simulink model "Control_try"  (R2021b)
settings: Solver=VariableStepAuto  StartTime=0.0  StopTime=inf  RelTol=1e-3
undefined symbols (not defined in the file or in its folder): DiscIntNeverNeededParam
libraries: mobileRoboticsLib x25, simulink_extras x1
(part 2 of 2)

== system Control_try/Team_1_behaviour/Goal_Keeper/min_Distance_Finder/Distance ==
  R_1_loc : Inport
  R_2_loc : Inport  Port=2
  Demux : Demux  Outputs=3
  Demux1 : Demux  Outputs=3
  Square : Math  Operator=square  SaturateOnIntegerOverflow=on
  Square Root : Sqrt  SaturateOnIntegerOverflow=on
  Square1 : Math  Operator=square  SaturateOnIntegerOverflow=on
  Sum : Sum  Inputs=|+-
  Sum1 : Sum  Inputs=|+-
  Sum2 : Sum  Inputs=|++
  R1_R2_dis : Outport
  wires:
  Square1/1 -> Sum2/2
  Demux/2 -> Sum1/1
  Sum2/1 -> Square Root/1
  Square/1 -> Sum2/1
  Demux/1 -> Sum/1
  Sum1/1 -> Square1/1
  Demux1/2 -> Sum1/2
  Sum/1 -> Square/1
  Demux1/1 -> Sum/2
  R_1_loc/1 -> Demux/1
  R_2_loc/1 -> Demux1/1
  Square Root/1 -> R1_R2_dis/1

== system Control_try/Team_1_behaviour/Goal_Keeper/min_Distance_Finder/Distance1 ==
  R_1_loc : Inport
  R_3_loc : Inport  Port=2
  Demux : Demux  Outputs=3
  Demux1 : Demux  Outputs=3
  Square : Math  Operator=square  SaturateOnIntegerOverflow=on
  Square Root : Sqrt  SaturateOnIntegerOverflow=on
  Square1 : Math  Operator=square  SaturateOnIntegerOverflow=on
  Sum : Sum  Inputs=|+-
  Sum1 : Sum  Inputs=|+-
  Sum2 : Sum  Inputs=|++
  R1_R3_dis : Outport
  wires:
  Square1/1 -> Sum2/2
  Demux/2 -> Sum1/1
  Sum2/1 -> Square Root/1
  Square/1 -> Sum2/1
  Demux/1 -> Sum/1
  Sum1/1 -> Square1/1
  Demux1/2 -> Sum1/2
  Sum/1 -> Square/1
  Demux1/1 -> Sum/2
  R_1_loc/1 -> Demux/1
  R_3_loc/1 -> Demux1/1
  Square Root/1 -> R1_R3_dis/1

== system Control_try/Team_1_behaviour/Goal_Keeper/min_Distance_Finder/Distance2 ==
  R_1_loc : Inport
  R_4_loc : Inport  Port=2
  Demux : Demux  Outputs=3
  Demux1 : Demux  Outputs=3
  Square : Math  Operator=square  SaturateOnIntegerOverflow=on
  Square Root : Sqrt  SaturateOnIntegerOverflow=on
  Square1 : Math  Operator=square  SaturateOnIntegerOverflow=on
  Sum : Sum  Inputs=|+-
  Sum1 : Sum  Inputs=|+-
  Sum2 : Sum  Inputs=|++
  R1_R4_dis : Outport
  wires:
  Square1/1 -> Sum2/2
  Demux/2 -> Sum1/1
  Sum2/1 -> Square Root/1
  Square/1 -> Sum2/1
  Demux/1 -> Sum/1
  Sum1/1 -> Square1/1
  Demux1/2 -> Sum1/2
  Sum/1 -> Square/1
  Demux1/1 -> Sum/2
  R_1_loc/1 -> Demux/1
  R_4_loc/1 -> Demux1/1
  Square Root/1 -> R1_R4_dis/1

== system Control_try/Team_1_behaviour/Goal_Keeper/min_Distance_Finder/R2_O_dist_val ==
  R_1_loc : Inport
  R_2_loc : Inport  Port=2
  sen_1_val : Inport  Port=3
  Chart : Stateflow chart  TreatAsAtomicUnit=on
  y : Outport
  wires:
  sen_1_val/1 -> Chart/2(sen_1_val)
  R_1_loc/1 -> Chart/1(R_1_loc)
  R_2_loc/1 -> Chart/3(R_2_loc)
  Chart/1(dist) -> y/1

== system Control_try/Team_1_behaviour/Goal_Keeper/min_Distance_Finder/R3_O_dist_val ==
  R_1_loc : Inport
  R_2_loc : Inport  Port=2
  sen_1_val : Inport  Port=3
  Chart : Stateflow chart  TreatAsAtomicUnit=on
  y : Outport
  wires:
  Chart/1(dist) -> y/1
  R_2_loc/1 -> Chart/3(R_2_loc)
  R_1_loc/1 -> Chart/1(R_1_loc)
  sen_1_val/1 -> Chart/2(sen_1_val)

== system Control_try/Team_1_behaviour/Goal_Keeper/min_Distance_Finder/R4_O_dist_val ==
  R_1_loc : Inport
  R_2_loc : Inport  Port=2
  sen_1_val : Inport  Port=3
  Chart : Stateflow chart  TreatAsAtomicUnit=on
  y : Outport
  wires:
  sen_1_val/1 -> Chart/2(sen_1_val)
  R_1_loc/1 -> Chart/1(R_1_loc)
  R_2_loc/1 -> Chart/3(R_2_loc)
  Chart/1(dist) -> y/1

== system Control_try/Team_1_behaviour/Roobot_2/min_Distance_Finder/Distance1 ==
  R_1_loc : Inport
  R_3_loc : Inport  Port=2
  Demux : Demux  Outputs=3
  Demux1 : Demux  Outputs=3
  Square : Math  Operator=square  SaturateOnIntegerOverflow=on
  Square Root : Sqrt  SaturateOnIntegerOverflow=on
  Square1 : Math  Operator=square  SaturateOnIntegerOverflow=on
  Sum : Sum  Inputs=|+-
  Sum1 : Sum  Inputs=|+-
  Sum2 : Sum  Inputs=|++
  R1_R3_dis : Outport
  wires:
  Square1/1 -> Sum2/2
  Demux/2 -> Sum1/1
  Sum2/1 -> Square Root/1
  Square/1 -> Sum2/1
  Demux/1 -> Sum/1
  Sum1/1 -> Square1/1
  Demux1/2 -> Sum1/2
  Sum/1 -> Square/1
  Demux1/1 -> Sum/2
  R_1_loc/1 -> Demux/1
  R_3_loc/1 -> Demux1/1
  Square Root/1 -> R1_R3_dis/1

== system Control_try/Team_1_behaviour/Roobot_2/min_Distance_Finder/Distance2 ==
  R_1_loc : Inport
  R_4_loc : Inport  Port=2
  Demux : Demux  Outputs=3
  Demux1 : Demux  Outputs=3
  Square : Math  Operator=square  SaturateOnIntegerOverflow=on
  Square Root : Sqrt  SaturateOnIntegerOverflow=on
  Square1 : Math  Operator=square  SaturateOnIntegerOverflow=on
  Sum : Sum  Inputs=|+-
  Sum1 : Sum  Inputs=|+-
  Sum2 : Sum  Inputs=|++
  R1_R4_dis : Outport
  wires:
  Square1/1 -> Sum2/2
  Demux/2 -> Sum1/1
  Sum2/1 -> Square Root/1
  Square/1 -> Sum2/1
  Demux/1 -> Sum/1
  Sum1/1 -> Square1/1
  Demux1/2 -> Sum1/2
  Sum/1 -> Square/1
  Demux1/1 -> Sum/2
  R_1_loc/1 -> Demux/1
  R_4_loc/1 -> Demux1/1
  Square Root/1 -> R1_R4_dis/1

== system Control_try/Team_1_behaviour/Roobot_2/min_Distance_Finder/R2_O_dist_val ==
  R_1_loc : Inport
  R_2_loc : Inport  Port=2
  sen_1_val : Inport  Port=3
  Chart : Stateflow chart  TreatAsAtomicUnit=on
  y : Outport
  wires:
  sen_1_val/1 -> Chart/2(sen_1_val)
  R_1_loc/1 -> Chart/1(R_1_loc)
  R_2_loc/1 -> Chart/3(R_2_loc)
  Chart/1(dist) -> y/1

== system Control_try/Team_1_behaviour/Roobot_2/min_Distance_Finder/R3_O_dist_val ==
  R_1_loc : Inport
  R_2_loc : Inport  Port=2
  sen_1_val : Inport  Port=3
  Chart : Stateflow chart  TreatAsAtomicUnit=on
  y : Outport
  wires:
  Chart/1(dist) -> y/1
  R_2_loc/1 -> Chart/3(R_2_loc)
  R_1_loc/1 -> Chart/1(R_1_loc)
  sen_1_val/1 -> Chart/2(sen_1_val)

== system Control_try/Team_1_behaviour/Roobot_2/min_Distance_Finder/R4_O_dist_val ==
  R_1_loc : Inport
  R_2_loc : Inport  Port=2
  sen_1_val : Inport  Port=3
  Chart : Stateflow chart  TreatAsAtomicUnit=on
  y : Outport
  wires:
  sen_1_val/1 -> Chart/2(sen_1_val)
  R_1_loc/1 -> Chart/1(R_1_loc)
  R_2_loc/1 -> Chart/3(R_2_loc)
  Chart/1(dist) -> y/1

== stateflow chart Control_try/Team 1 Behaviour/kick_direction/Chart1 ==
  state x_pos
    du:
    Vx = 1
  state x_neg
    du:
    Vx = -1
  (default) -> x_pos
  x_pos -> x_neg : [x > 0]
  x_neg -> x_pos : [x<1]
  data: Vx output; x input

== stateflow chart Control_try/Team 1 Behaviour/kick_direction/Chart2 ==
  state y_pos
    du:
    Vy = 1
  state y_neg
    du:
    Vy = -1
  (default) -> y_pos
  y_pos -> y_neg : [y > 0]
  y_neg -> y_pos : [y<1]
  data: y input; Vy output

== stateflow chart Control_try/Team 1 Behaviour/Velocity_Decider ==
  state Robot_Far
    du:
    velocity = 1;
    kick = 0;
  state Robot_Close
    du:
    velocity = 0;
    kick = 1;
  (default) -> Robot_Far
  Robot_Far -> Robot_Close : [DBR <= 0.25]
  Robot_Close -> Robot_Far : [DBR > 0.25]
  data: kick output; DBR input; velocity output

== stateflow chart Control_try/Team 1 Behaviour/Chart ==
  state second_coordinate
    du:
    actual_angle = -pi +angle + angle_bot;
  state first_coordinate
    du:
    actual_angle = angle_bot - angle;
  state ffourth_coordinate
    du:
    actual_angle = -(2*pi) + angle + angle_bot
  state Third_coordinate
    du:
    actual_angle =-(pi) - angle + angle_bot;
  (default) -> first_coordinate
  first_coordinate -> second_coordinate [order 1] : [ Rx>Bx && Ry<By ]
  second_coordinate -> first_coordinate [order 1] : [ Rx<Bx && Ry<By]
  ffourth_coordinate -> second_coordinate [order 1] : [ Rx>Bx && Ry<By ]
  first_coordinate -> Third_coordinate [order 3] : [ Rx>Bx && Ry>By]
  second_coordinate -> Third_coordinate [order 3] : [ Rx>Bx && Ry>By ]
  Third_coordinate -> second_coordinate [order 1] : [ Rx>Bx && Ry<By ]
  second_coordinate -> ffourth_coordinate [order 2] : [ Rx<Bx && Ry>By ]
  Third_coordinate -> first_coordinate [order 2] : [ Rx<Bx && Ry<By ]
  ffourth_coordinate -> first_coordinate [order 2] : [ Rx<Bx && Ry<By ]
  first_coordinate -> ffourth_coordinate [order 2] : [ Rx<Bx && Ry>By ]
  Third_coordinate -> ffourth_coordinate [order 3] : [ Rx<Bx && Ry>By ]
  ffourth_coordinate -> Third_coordinate [order 3] : [ Rx>Bx && Ry>By]
  data: Bx input; By input; Rx input; Ry input; angle input; actual_angle output; angle_bot input

== stateflow chart Control_try/Team 1 Behaviour/Chart3 ==
  state stop
    du:
    w = 0;
    v=0.25 * velocity;
  state RCW
    du:
    w = -1*1;
    v=0;
  state RCCW
    du:
    w =1*1;
    v=0;
  (default) -> stop
  stop -> RCCW [order 2] : [after(1,sec) && DT > 0]
  stop -> RCW [order 1] : [after(1,sec) && DT < 0]
  RCW -> stop [order 1] : [DT<= 0.1 && DT>= -0.1]
  RCCW -> stop [order 1] : [DT<= 0.1 && DT>= -0.1]
  RCCW -> RCW [order 2] : [DT>0]
  RCW -> RCCW [order 2] : [DT<0]
  data: velocity input; v output; DT input; w output

== stateflow chart Control_try/Referee/GOAL ==
  state Start
    en:
    right_team_goal = 0;
    left_team_goal = 0;
  state Goal_left
    en:
    right_team_goal = right_team_goal +1 ;
  state in_field
    en:
  state Goal_right
    en:
    left_team_goal = left_team_goal + 1;
  (default) -> Start
  Start -> in_field : [X > 1 && X<10 && Y > 1  && Y < 7]
  in_field -> Goal_left [order 2] : [fix(X) == 1 && Y > 2.7  && Y < 5.3 && Z < 1.2]
  Goal_right -> in_field : [X > 1 && X<10 && Y > 1  && Y < 7]
  in_field -> Goal_right [order 1] : [fix(X) == 10 && Y > 2.7  && Y < 5.3 && Z <1.2]
  Goal_left -> in_field : [X > 1 && X<10 && Y > 1  && Y < 7]
  data: X input; Y input; Z input; left_team_goal output; right_team_goal output

== stateflow chart Control_try/Referee/Throwin ==
  data: X input; Y input

== stateflow chart Control_try/Referee/Corner ==

== stateflow chart Control_try/Referee/Penelty ==

== matlab function Control_try/Enviornment/MATLAB Function ==

function plotEnvironment

coder.extrinsic('evalin');
persistent hasPlotted
if isempty(hasPlotted)
    evalin('base','environment_Plot');
    hasPlotted = true;
end

== stateflow chart Control_try/Enviornment/Ball_Dynamics/Chart ==
  state on_ground
    du:
    if(abs(F)>2.6)
    a = (abs(F)-2.6) * (F/abs(F)) / 0.43
    else
    a = 0
    end
  state off_ground
    du:
    a = F/0.43
  (default) -> on_ground
  off_ground -> on_ground : [Y ==0]
  on_ground -> off_ground : [Y > 0]
  data: Y input; F input; a output

== stateflow chart Control_try/Enviornment/Ball_Dynamics/Chart1 ==
  state calculations_neg
    du:
    vs = (abs(v))*(abs(v))*(-1)
  state calculations_pos
    du:
    vs = v*v
  (default) -> calculations_neg
  calculations_pos -> calculations_neg : [v<0]
  calculations_neg -> calculations_pos : [v>0]
  data: vs output; v input

== stateflow chart Control_try/Enviornment/Ball_Dynamics/Chart2 ==
  state on_ground
    du:
    if(abs(F)>2.6)
    a = (abs(F) - 2.6) * (F/abs(F)) / 0.43
    else
    a = 0
    end
  state off_ground
    du:
    a = F/0.43
  (default) -> on_ground
  off_ground -> on_ground : [Y ==0]
  on_ground -> off_ground : [Y > 0]
  data: Y input; F input; a output

== stateflow chart Control_try/Enviornment/Ball_Dynamics/Chart3 ==
  state calculations_neg
    du:
    vs = (abs(v))*(abs(v))*(-1)
  state calculations_pos
    du:
    vs = v*v
  (default) -> calculations_neg
  calculations_pos -> calculations_neg : [v<0]
  calculations_neg -> calculations_pos : [v>=0]
  data: vs output; v input

== stateflow chart Control_try/Enviornment/Ball_Dynamics/Chart4 ==
  state in_motion
    du:
    if (v > 0)
    a = -(0.32*0.98)
    else if(v<0)
    a = (0.32*0.98)
    end
    end
  state stationary
    du:
    a = 0;
  (default) -> in_motion
  in_motion -> stationary : [abs(v) < 0.03 | Y>0]
  stationary -> in_motion : [abs(v)>0.03]
  data: Y input; a output; v input

== stateflow chart Control_try/Team_1_behaviour/Goal_Keeper/control ==
  state Ball_Following
    du:
    kick = 0;
    if (R1_loc_Y>2.7 && R1_loc_Y<5.3)
    if(Ball_loc_Y > R1_loc_Y)
    R1_vel_Y = 0.1;
    else if (Ball_loc_Y < R1_loc_Y)
    R1_vel_Y = -0.1;
    end
    end
    else if ( R1_loc_Y > 5.3)
    R1_vel_Y = -0.1;
    else if ( R1_loc_Y < 2.7)
    R1_vel_Y = -0.1;
    end
    end
    end
  state Ball_Held
    du:
    kick = 1;
  (default) -> Ball_Following
  Ball_Following -> Ball_Held : [GB_dist < 0.25]
  Ball_Held -> Ball_Following : [GB_dist > 0.25]
  data: kick output; R1_loc_X input; Ball_loc_X input; GB_dist input; R1_loc_Y input; Ball_loc_Y input; R1_vel_Y output

== stateflow chart Control_try/Enviornment/Ball_Dynamics/Chart6 ==
  state in_motion
    du:
    if (v > 0)
    a = -(0.32*0.98)
    else if(v<0)
    a = (0.32*0.98)
    end
    end
  state stationary
    du:
    a = 0;
  (default) -> in_motion
  in_motion -> stationary : [abs(v) < 0.01 | Y>0]
  stationary -> in_motion : [abs(v)>0.02]
  data: Y input; a output; v input

== stateflow chart Control_try/Team_1_behaviour/Goal_Keeper/min_Distance_Finder/Kick_prob_calc ==
  state bot_2
    du:
    kick_direction = R_2_loc
  state bot_3
    du:
    kick_direction = R_3_loc
  state bot_4
    du:
    kick_direction = R_4_loc
  (default) -> bot_2
  bot_2 -> bot_3 [order 1] : [R1_R3_dis < R1_R2_dis && R1_R3_dis < R1_R4_dis]
  bot_3 -> bot_2 [order 1] : [R1_R2_dis < R1_R3_dis && R1_R2_dis < R1_R4_dis]
  bot_4 -> bot_2 [order 2] : [R1_R2_dis < R1_R3_dis && R1_R2_dis < R1_R4_dis]
  bot_2 -> bot_4 [order 2] : [R1_R4_dis < R1_R3_dis && R1_R4_dis < R1_R2_dis]
  bot_3 -> bot_4 [order 2] : [R1_R4_dis < R1_R3_dis && R1_R4_dis < R1_R2_dis]
  bot_4 -> bot_3 [order 1] : [R1_R3_dis < R1_R2_dis && R1_R3_dis < R1_R4_dis]
  data: R_4_loc input; R_2_loc input; R_3_loc input; R1_R2_dis input; R1_R3_dis input; R1_R4_dis input; kick_direction output

== stateflow chart Control_try/Team_1_behaviour/Goal_Keeper/min_Distance_Finder/R3_O_dist_val/Chart ==
  state calculate
    en:
    dist = 0;
    pos_x = 0;
    pos_y =0;
    dist_x =0;
    dist_y = 0;
    i=0;
    du:
    dist = 0;
    for i=1:7
    if (sen_1_val(i,3) > 4)
    pos_x = R_1_loc(1) + sen_1_val(i,1);
    pos_y = R_1_loc(2) + sen_1_val(i,2);
    dist_x = R_2_loc(1) - pos_x;
    dist_y = R_2_loc(2) - pos_y;
    dist = dist + sqrt((dist_x*dist_x) + (dist_y*dist_y));
    end
    end
  (default) -> calculate
  data: R_1_loc input; sen_1_val input; dist output; R_2_loc input; dist_y local; i local; pos_x local; pos_y local; dist_x local

== stateflow chart Control_try/Team_1_behaviour/Goal_Keeper/min_Distance_Finder/R2_O_dist_val/Chart ==
  state calculate
    en:
    dist = 0;
    pos_x = 0;
    pos_y =0;
    dist_x =0;
    dist_y = 0;
    i=0;
    du:
    dist = 0;
    for i=1:7
    if (sen_1_val(i,3) > 4)
    pos_x = R_1_loc(1) + sen_1_val(i,1);
    pos_y = R_1_loc(2) + sen_1_val(i,2);
    dist_x = R_2_loc(1) - pos_x;
    dist_y = R_2_loc(2) - pos_y;
    dist = dist + sqrt((dist_x*dist_x) + (dist_y*dist_y));
    end
    end
  (default) -> calculate
  data: R_1_loc input; sen_1_val input; dist output; R_2_loc input; dist_y local; i local; pos_x local; pos_y local; dist_x local

== stateflow chart Control_try/Team_1_behaviour/Goal_Keeper/min_Distance_Finder/R4_O_dist_val/Chart ==
  state calculate
    en:
    dist = 0;
    pos_x = 0;
    pos_y =0;
    dist_x =0;
    dist_y = 0;
    i=0;
    du:
    dist = 0;
    for i=1:7
    if (sen_1_val(i,3) > 4)
    pos_x = R_1_loc(1) + sen_1_val(i,1);
    pos_y = R_1_loc(2) + sen_1_val(i,2);
    dist_x = R_2_loc(1) - pos_x;
    dist_y = R_2_loc(2) - pos_y;
    dist = dist + sqrt((dist_x*dist_x) + (dist_y*dist_y));
    end
    end
  (default) -> calculate
  data: R_1_loc input; sen_1_val input; dist output; R_2_loc input; dist_y local; i local; pos_x local; pos_y local; dist_x local

== stateflow chart Control_try/Team_1_behaviour/Goal_Keeper/kick_direction/Chart1 ==
  state x_pos
    du:
    Vx = 1
  state x_neg
    du:
    Vx = -1
  (default) -> x_pos
  x_pos -> x_neg : [x > 0]
  x_neg -> x_pos : [x<1]
  data: Vx output; x input

== stateflow chart Control_try/Team_1_behaviour/Goal_Keeper/kick_direction/Chart2 ==
  state y_pos
    du:
    Vy = 1
  state y_neg
    du:
    Vy = -1
  (default) -> y_pos
  y_pos -> y_neg : [y > 0]
  y_neg -> y_pos : [y<1]
  data: y input; Vy output

== stateflow chart Control_try/Enviornment/kick_director/Chart ==
  state P1_kick
    du:
    KF = [p1(1);p1(2);p1(3);p1(4)]
    bot_tag = 1
  state P5_kick
    du:
    KF = p5
    bot_tag = 5
  state no_ball_kick
    du:
    KF = [0;0;0;0]
  state P2_kick
    du:
    KF = p2
    bot_tag = 2
  state P6_kick
    du:
    KF = p6
    bot_tag = 6
  state P3_kick
    du:
    KF = p3
    bot_tag = 3
  state P7_kick
    du:
    KF = p7
    bot_tag = 7
  state P4_kick
    du:
    KF = p4
    bot_tag = 4
  state P8_kick
    du:
    KF = p8
    bot_tag = 8
  (default) -> no_ball_kick
  P5_kick -> no_ball_kick : [p5(4) == 0]
  no_ball_kick -> P5_kick [order 5] : [p5(4) == 1]
  P1_kick -> no_ball_kick : [p1(4) == 0]
  no_ball_kick -> P1_kick [order 1] : [p1(4) == 1]
  no_ball_kick -> P2_kick [order 2] : [p2(4) == 1]
  no_ball_kick -> P6_kick [order 6] : [p6(4) == 1]
  P2_kick -> no_ball_kick : [p2(4) == 0]
  P6_kick -> no_ball_kick : [p6(4) == 0]
  P3_kick -> no_ball_kick : [p3(4) == 0]
  P7_kick -> no_ball_kick : [p7(4) == 0]
  no_ball_kick -> P7_kick [order 7] : [p7(4) == 1]
  no_ball_kick -> P3_kick [order 3] : [p3(4) == 1]
  no_ball_kick -> P8_kick [order 8] : [p8(4) == 1]
  no_ball_kick -> P4_kick [order 4] : [p4(4) == 1]
  P4_kick -> no_ball_kick : [p4(4) == 0]
  P8_kick -> no_ball_kick : [p8(4) == 0]
  data: bot_tag output; p1 input; p2 input; p3 input; p4 input; p5 input; p6 input; p7 input; p8 input; KF output

== matlab function Control_try/Team_1_behaviour/Goal_Keeper/min_Distance_Finder/zero_padding ==
  data: u input; y output
function y = pad(u)
% Zero-pads object detections to work with arrays of buses

y = zeros(7,3);
numElems = min(size(u,1),7);
for idx = 1:numElems
   y(idx,1:3) = u(idx,1:3); 
end
end

== matlab function Control_try/Team_1_behaviour/Goal_Keeper/MATLAB Function ==
  data: robotLoc input; newHeadingAngle output; checkpoint input
function newHeadingAngle  = ComputeHeadingAngle(robotLoc, checkpoint)

currentLocation = [robotLoc(1),robotLoc(2)];

deltaPosition = checkpoint - currentLocation;

calculatedHeadingAngle = atan2( deltaPosition(1), deltaPosition(2) );

if isnan(calculatedHeadingAngle)
    if deltaPosition(2) >= 0
        newHeadingAngle = pi/2;
    else
        newHeadingAngle = -pi/2;
    end
else
    newHeadingAngle = calculatedHeadingAngle;
end

end

== stateflow chart Control_try/Team_1_behaviour/Roobot_2/control ==
  state Ball_Following
    en,du:
    distance_to_ball = Distance(R2_loc (1), R2_loc (2), Ball_loc_X,Ball_loc_Y);
    ball_loc = [Ball_loc_X,Ball_loc_Y];
    %angle = ComputeHeadingAngle(R2_loc,ball_loc,0.05);
    [x_res, y_res] = velocityResolver(angle);
    distance_to_goal = Distance(R2_loc(1),R2_loc(2),10,4);
    if(distance_to_ball<0.15)
    pass_beh = pass_behaviour_controller(distance_to_goal,nearest_op,nearest_team);
    %kick =1;
    %else
    %move_to_ball;
    %R2_vel_X = 0.44 * x_res;
    %R2_vel_Y = 0.44 *y_res;
    %R1_vel_X = 03. * resolver(1);
    %R1_vel_Y = 0.3 * resolver(2);
    %R1_vel_X = 0.12 * resolver(1);
    %R1_vel_Y = 0.12 * resolver(2);
    end
  state Shoot
    en,du:
    distance_to_goal_1 = Distance(10,3.35,R2_loc(1),R2_loc(2));
    distance_to_goal_2 = Distance(10,4.65,R2_loc(1),R2_loc(2));
    shoot_region = shooting_spot_rev1_controller(distance_to_goal_1,GoalKeeperY,distance_to_goal_2);
    kick_angle = ComputeKickingAngle(R2_loc, [10,shoot_region]);
    kick = 1;
  state dribble
    du:
    R2_vel_X = 0;
    R2_vel_Y = 0;
  state pass
    kick_angle = ComputeKickingAngle(R2_loc, nearest_robot);
  (default) -> Ball_Following
  Shoot -> Ball_Following : [after(1,sec)]
  Ball_Following -> dribble [order 2] : [pass_beh == 2]
  dribble -> Ball_Following : [after(1,sec)]
  Ball_Following -> Shoot [order 1] : [pass_beh == 3]
  Ball_Following -> pass [order 3] : [pass_beh == 1]
  pass -> Ball_Following : [after(1,sec)]
  data: angle1 function_input; vx function_output; vy function_output; ball_distance function_input; ball_velocity function_input; movement function_output; distancetogoal function_input; nearest_oponent_distance function_input; nearest_team_player_distance function_input; pass_behaviour function_output; distance_to_goal1 function_input; goal_keeperY function_input; distance_to_goal2 function_input; centroid function_output; robotLoc function_input; checkpoint function_input; newHeadingAngle function_output; tolerance function_input; x1 function_input; y1 function_input; x2 function_input; y2 function_input; distance function_output; robotLoc function_input; checkpoint function_input; newHeadingAngle function_output; kick output; R2_loc input; Ball_loc_X input; GB_dist input; Ball_loc_Y input; R2_vel_Y output =0; ball_vel_x input; ball_vel_y input; GoalKeeperY input; distance_to_ball local; distance_to_goal_1 local; distance_to_goal_2 local; resolver local; shoot_region local; distance_to_goal local; R2_vel_X output =0; nearest_team input; nearest_team_idx input; nearest_op input; kick_angle output; pass_beh local =0; nearest_robot input; y_res local; x_res local; angle output =0; ball_loc local
  function [vx,vy] = velocityResolver(angle1):
    | function [vx,vy] = velocityResolver(angle1)
    | 
    | vx = cos(angle1);
    | vy = sin(angle1);
    | 
    | end
  function movement  = robot_moving_speed_controller(ball_distance, ball_velocity):
    | function movement  = robot_moving_speed_controller(ball_distance, ball_velocity)
    | %UNTITLED2 Summary of this function goes here
    | %   Detailed explanation goes here
    | MovingSpeedFuzzyFile= readfis('robot_moving_speed');
    | A = evalfis(MovingSpeedFuzzyFile,[ball_distance, ball_velocity]);
    | if ( A(1)<0.5 )
    | movement=1;
    | elseif ( 0.5<=A(2) && A(2)<2.5 )
    | movement=2;
    | elseif ( A(3)>2.5 )
    | movement=3;
    | end
    | 
    | end
  function pass_behaviour  = pass_behaviour_controller(distancetogoal,nearest_oponent_distance,nearest_team_player_distance):
    | function pass_behaviour  = pass_behaviour_controller(distancetogoal,nearest_oponent_distance,nearest_team_player_distance)
    | %PASS_BEHAVIOR Summary of this function goes here
    | %   Detailed explanation goes here
    | behaviourFuzzyFile= getFISCodeGenerationData('pass_behaviour.fis');
    | b = evalfis(behaviourFuzzyFile,[distancetogoal,nearest_oponent_distance,nearest_team_player_distance]);
    | 
    | if ( b<0.4 )
    | pass_behaviour=1;
    | elseif ( 0.4<=b && b<0.6 )
    | pass_behaviour=2;
    | else
    | pass_behaviour=3;
    | end
    | 
    | end
  function centroid  = shooting_spot_rev1_controller(distance_to_goal1, goal_keeperY, distance_to_goal2):
    | function centroid  = shooting_spot_rev1_controller(distance_to_goal1, goal_keeperY, distance_to_goal2)
    | %UNTITLED3 Summary of this function goes here
    | %   Detailed explanation goes here
    | ShootingSpotFuzzyFile= getFISCodeGenerationData('shooting_spot_rev1');
    | C = evalfis(ShootingSpotFuzzyFile,[distance_to_goal1, goal_keeperY, distance_to_goal2]);
    | if ( C<1 )
    | % shooting_region=1;
    | centroid = [4.65,0.3];
    | elseif ( 1<=C && C<2 )
    | % shooting_region=2;
    | centroid = [3.35,0.3];
    | elseif ( 2<=C && C<3 )
    | % shooting_region=3;
    | centroid = [4.65,0.9];
    | else
    | % shooting_region=4;
    | centroid = [3.35,0.9];
    | end
    | end
  function newHeadingAngle  = ComputeHeadingAngle(robotLoc, checkpoint,tolerance):
    | function newHeadingAngle  = ComputeHeadingAngle(robotLoc, checkpoint,tolerance)
    | 
    | currentLocation = [robotLoc(1),robotLoc(2)];
    | 
    | 
    | % Check to see if within tolerance 
    | deltaPosition = checkpoint - currentLocation;
    | distanceFromCheckpoint = norm(deltaPosition);
    | 
    | booleanAtCheckpoint = (distanceFromCheckpoint < tolerance);
    | 
    | % Calculate new heading
    | calculatedHeadingAngle = atan2( deltaPosition(2), deltaPosition(1) );
    | 
    | if isnan(calculatedHeadingAngle)
    |     if deltaPosition(2) >= 0
    |         newHeadingAngle = pi/2;
    |     else
    |         newHeadingAngle = -pi/2;
    |     end
    | else
    |     newHeadingAngle = calculatedHeadingAngle;
    | end
    | 
    | end
  function distance = Distance(x1,y1,x2,y2):
    | function distance = Distance(x1,y1,x2,y2)
    | distance = sqrt((x1-x2).^2 + (y1 +y2).^2);
    | end
  function newHeadingAngle  = ComputeKickingAngle(robotLoc, checkpoint):
    | function newHeadingAngle  = ComputeKickingAngle(robotLoc, checkpoint)
    | 
    | currentLocation = [robotLoc(1),robotLoc(2),0];
    | 
    | deltaPosition = checkpoint - currentLocation;
    | 
    | calculatedHeadingAngle = atan2( deltaPosition(2), deltaPosition(1));
    | 
    | if isnan(calculatedHeadingAngle)
    |     if deltaPosition(1) >= 0
    |         newHeadingAngle = pi/2;
    |     else
    |         newHeadingAngle = -pi/2;
    |     end
    | else
    |     newHeadingAngle = calculatedHeadingAngle;
    | end
    | 
    | end

== matlab function Control_try/Team_1_behaviour/Roobot_2/min_Distance_Finder/MATLAB Function ==
  data: min input; y output; rob3 input
function y = fcn(min, rob3)
 if min == rob3
y = 3;
 else 
     y =4;
 end
end

== stateflow chart Control_try/Team_1_behaviour/Roobot_2/min_Distance_Finder/R2_O_dist_val/Chart ==
  state calculate
    en:
    dist = 0;
    pos_x = 0;
    pos_y =0;
    dist_x =0;
    dist_y = 0;
    i=0;
    du:
    dist = 0;
    for i=1:7
    if (sen_1_val(i,3) > 4)
    pos_x = R_1_loc(1) + sen_1_val(i,1);
    pos_y = R_1_loc(2) + sen_1_val(i,2);
    dist_x = R_2_loc(1) - pos_x;
    dist_y = R_2_loc(2) - pos_y;
    dist = dist + sqrt((dist_x*dist_x) + (dist_y*dist_y));
    end
    end
  (default) -> calculate
  data: R_1_loc input; sen_1_val input; dist output; R_2_loc input; dist_y local; i local; pos_x local; pos_y local; dist_x local

== stateflow chart Control_try/Team_1_behaviour/Roobot_2/min_Distance_Finder/R3_O_dist_val/Chart ==
  state calculate
    en:
    dist = 0;
    pos_x = 0;
    pos_y =0;
    dist_x =0;
    dist_y = 0;
    i=0;
    du:
    dist = 0;
    for i=1:7
    if (sen_1_val(i,3) > 4)
    pos_x = R_1_loc(1) + sen_1_val(i,1);
    pos_y = R_1_loc(2) + sen_1_val(i,2);
    dist_x = R_2_loc(1) - pos_x;
    dist_y = R_2_loc(2) - pos_y;
    dist = dist + sqrt((dist_x*dist_x) + (dist_y*dist_y));
    end
    end
  (default) -> calculate
  data: R_1_loc input; sen_1_val input; dist output; R_2_loc input; dist_y local; i local; pos_x local; pos_y local; dist_x local

== stateflow chart Control_try/Team_1_behaviour/Roobot_2/min_Distance_Finder/R4_O_dist_val/Chart ==
  state calculate
    en:
    dist = 0;
    pos_x = 0;
    pos_y =0;
    dist_x =0;
    dist_y = 0;
    i=0;
    du:
    dist = 0;
    for i=1:7
    if (sen_1_val(i,3) > 4)
    pos_x = R_1_loc(1) + sen_1_val(i,1);
    pos_y = R_1_loc(2) + sen_1_val(i,2);
    dist_x = R_2_loc(1) - pos_x;
    dist_y = R_2_loc(2) - pos_y;
    dist = dist + sqrt((dist_x*dist_x) + (dist_y*dist_y));
    end
    end
  (default) -> calculate
  data: R_1_loc input; sen_1_val input; dist output; R_2_loc input; dist_y local; i local; pos_x local; pos_y local; dist_x local

== matlab function Control_try/Team_1_behaviour/Roobot_2/min_Distance_Finder/zero_padding ==
  data: u input; y output
function y = pad(u)
% Zero-pads object detections to work with arrays of buses

y = zeros(7,3);
numElems = min(size(u,1),7);
for idx = 1:numElems
   y(idx,1:3) = u(idx,1:3); 
end
end

== matlab function Control_try/MATLAB Function ==
  data: F input; dF output; dis input; dT input
function dF = fcn(F,dis,dT)


F_x_max = max(abs(F(:,1))) ;
F_y_max = max(abs(F(:,2))) ;

Fmax = sqrt((F_x_max^2)+(F_y_max^2)) ;

fc = sqrt(2*dis*dis*dT) ;

if fc <= Fmax
    dF = fc ;
else
    dF = Fmax ;
end

end

== stateflow chart Control_try/Team_1_behaviour/Roobot_2/Chart ==
  state stop
    du:
    w = 0;
  state RCW
    du:
    w = -1*0.1;
  state RCCW
    du:
    w =1*0.1;
  (default) -> stop
  stop -> RCCW [order 2] : [angle_to_turn > 0]
  stop -> RCW [order 1] : [angle_to_turn < 0]
  RCW -> stop [order 1] : [angle_to_turn<= 0.3 && angle_to_turn>= -0.3]
  RCCW -> stop [order 1] : [angle_to_turn<= 0.3 && angle_to_turn>= -0.3]
  RCCW -> RCW [order 2] : [angle_to_turn>0]
  RCW -> RCCW [order 2] : [angle_to_turn<0]
  data: w output; angle_to_turn input

== matlab function Control_try/Team_1_behaviour/Roobot_2/MATLAB Function ==
  data: robotLoc input; newHeadingAngle output; checkpoint input
function newHeadingAngle  = ComputeHeadingAngle(robotLoc, checkpoint)

currentLocation = [robotLoc(1),robotLoc(2)];
ball_location = [checkpoint(1),checkpoint(2)];
tolerance  = 0.05;

% Check to see if within tolerance 
deltaPosition = ball_location - currentLocation;
distanceFromCheckpoint = norm(deltaPosition);

booleanAtCheckpoint = (distanceFromCheckpoint < tolerance);

% Calculate new heading
calculatedHeadingAngle = atan2( deltaPosition(2), deltaPosition(1) );

if isnan(calculatedHeadingAngle)
    if deltaPosition(2) >= 0
        newHeadingAngle = pi/2;
    else
        newHeadingAngle = -pi/2;
    end
else
    newHeadingAngle = calculatedHeadingAngle;
end

end

== matlab function Control_try/Team_1_behaviour/Roobot_2/MATLAB Function1 ==
  data: u input; y output; v input
function y = fcn(u,v)

y = -angdiff(u,v);
end

== stateflow chart Control_try/Team_1_behaviour/Roobot_2/Chart1 ==
  state second_coordinate
    du:
    actual_angle = -pi +angle + angle_bot;
  state first_coordinate
    du:
    actual_angle = angle_bot - angle;
  state ffourth_coordinate
    du:
    actual_angle = -(2*pi) + angle + angle_bot
  state Third_coordinate
    du:
    actual_angle =-(pi) - angle + angle_bot;
  (default) -> first_coordinate
  first_coordinate -> second_coordinate [order 1] : [ Rx>Bx && Ry<By ]
  second_coordinate -> first_coordinate [order 1] : [ Rx<Bx && Ry<By]
  ffourth_coordinate -> second_coordinate [order 1] : [ Rx>Bx && Ry<By ]
  first_coordinate -> Third_coordinate [order 3] : [ Rx>Bx && Ry>By]
  second_coordinate -> Third_coordinate [order 3] : [ Rx>Bx && Ry>By ]
  Third_coordinate -> second_coordinate [order 1] : [ Rx>Bx && Ry<By ]
  second_coordinate -> ffourth_coordinate [order 2] : [ Rx<Bx && Ry>By ]
  Third_coordinate -> first_coordinate [order 2] : [ Rx<Bx && Ry<By ]
  ffourth_coordinate -> first_coordinate [order 2] : [ Rx<Bx && Ry<By ]
  first_coordinate -> ffourth_coordinate [order 2] : [ Rx<Bx && Ry>By ]
  Third_coordinate -> ffourth_coordinate [order 3] : [ Rx<Bx && Ry>By ]
  ffourth_coordinate -> Third_coordinate [order 3] : [ Rx>Bx && Ry>By]
  data: Bx input; By input; Rx input; Ry input; angle input; actual_angle output; angle_bot input

== matlab function Control_try/Team_1_behaviour/Roobot_2/MATLAB Function2 ==
  data: robotLoc input; newHeadingAngle output; ballLoc input; tolerance input
function newHeadingAngle  = ComputeHeadingAngle(robotLoc, ballLoc,tolerance)

currentLocation = [robotLoc(1),robotLoc(2)];
checkpoint = [ballLoc(1),ballLoc(2)];

% Check to see if within tolerance 
deltaPosition = checkpoint - currentLocation;
distanceFromCheckpoint = norm(deltaPosition);

booleanAtCheckpoint = (distanceFromCheckpoint < tolerance);

% Calculate new heading
calculatedHeadingAngle = atan2( deltaPosition(2), deltaPosition(1) );

if isnan(calculatedHeadingAngle)
    if deltaPosition(2) >= 0
        newHeadingAngle = pi/2;
    else
        newHeadingAngle = -pi/2;
    end
else
    newHeadingAngle = calculatedHeadingAngle;
end

end
